simulink model "auv_modell_camsim_kalman"  (Simulink 7.0)
settings: Solver=ode4  StartTime=0.0  StopTime=100  FixedStep=0.1  RelTol=1e-3
values from neighbouring files (symbols this model uses):
  eta0 = [0 0 0 0 0 0]'    [initauv.m]
undefined symbols (not defined in the file or in its folder): C_calc, ekf
libraries: marine_gnc x2, fordypningsprosjekt x1, simulink x1
settings Model: Creator=anderga  LastModifiedBy=anderga  ExtModeAutoUpdateStatusClock=off  BufferReuse=off
settings OptimizationCC: BlockReduction=off  InlineParams=on  BufferReuse=off

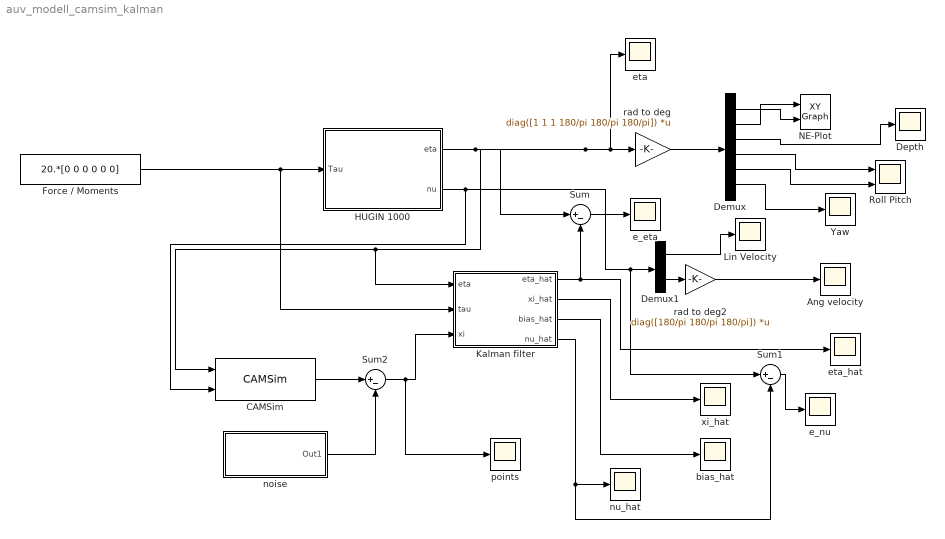
== system auv_modell_camsim_kalman ==
  Ang velocity : Scope
      settings: YMin=-1  YMax=1  SaveName=ScopeData6
  CAMSim : fordypningsprosjekt/CAMSim  SystemSampleTime=-1
  Demux : Demux  Outputs=6
  Demux1 : Demux  Outputs=2
  Depth : Scope
      settings: TimeRange=400  YMin=-140  YMax=40  SaveName=ScopeData4
  Force / Moments : Constant  Value=20.*[0 0 0 0 0 0]  OutDataType=sfix(16)  OutScaling=2^0
  HUGIN 1000 : Subsystem  mask(HUGIN 1000 AUV){eta_0=eta0, nu_0=[0 0 0 0 0 0]}
      mask prompts: eta_0 "Initial Position [x y z phi theta psi]"; nu_0 "Initial speed [u v w p q r]"
      mask help:
      | The hydrodynamic model of Kongsberg Maritimes
      | AUV type HUGIN 1000.
      |
      | Implemented using
      |
      | eta_dot = J(eta)*nu
      | M*nu_dot + C(nu)*nu + D(nu)*nu + g(eta) = tau
      |
      | and the MMS toolbox from www.marinecybernetics.org
      mask init:
      | m = 1380;
      | xg = 0;
      | yg = 0;
      | zg = 0.0328;
      | Ix = 86.53;
      | Iy = 1247;
      | Iz = 1247;
      | 
      | Xu = -85.57;
      | Yv = -1092.9;
      | Yr = -84.1448;
      | Zw = -1092.9;
      | Zq = 84.1448;
      | Mq = -795.1686;
      | Nr = -795.1686;
      |     
      | M = [m-Xu   0       0       0       m*zg    -m*yg;
      |      0      m-Yv    0       -m*zg   0       m*xg-Yr;
      |      0      0       m-Zw    m*yg    -m*xg-Zq 0;
      |      0      -m*zg   m*yg    Ix      0        0;
      |      m*zg   0       -m*xg-Zq 0      Iy-Mq    0;
      |      -m*yg  m*xg-Yr 0       0       0       Iz-Nr];
  Kalman filter : Subsystem
  Lin Velocity : Scope
      settings: YMin=-0.05  YMax=0.65
  NE-Plot : simulink/Sinks/XY Graph  SystemSampleTime=-1  xmin=-100  xmax=220  ymin=-100  ymax=1000  st=-1
  Roll Pitch : Scope  NumInputPorts=2
      settings: TimeRange=400  YMin=-1~-0.25  YMax=1~0  SaveName=ScopeData3
  Sum : Sum  Inputs=|+-  OutDataType=sfix(16)  OutScaling=2^0
  Sum1 : Sum  Inputs=|+-  OutDataType=sfix(16)  OutScaling=2^0
  Sum2 : Sum  Inputs=|+-  OutDataType=sfix(16)  OutScaling=2^0
  Yaw : Scope
      settings: TimeRange=100  YMin=1  YMax=4.75  SaveName=ScopeData2
  bias_hat : Scope
      settings: YMin=-0.015  YMax=0.001  SaveName=ScopeData11
  e_eta : Scope
      settings: TimeRange=100  YMin=-0.0007  YMax=5e-005  SaveName=ScopeData14
  e_nu : Scope
      settings: YMin=-0.25  YMax=2.75  SaveName=ScopeData15
  eta : Scope
      settings: YMax=6
  eta_hat : Scope
      settings: YMin=-80  YMax=10  SaveName=ScopeData9
  noise : Subsystem
  nu_hat : Scope
      settings: YMin=-200  YMax=25  SaveName=ScopeData12
  points : Scope
      settings: TimeRange=100  YMin=-7  YMax=7  SaveName=ScopeData13
  rad to deg : Gain  Gain=diag([1 1 1 180/pi 180/pi 180/pi])  Multiplication=Matrix(K*u)  ParameterDataType=sfix(16)  ParameterScaling=2^0  OutDataType=sfix(16)  OutScaling=2^0
  rad to deg2 : Gain  Gain=diag([180/pi 180/pi 180/pi])  Multiplication=Matrix(K*u)  ParameterDataType=sfix(16)  ParameterScaling=2^0  OutDataType=sfix(16)  OutScaling=2^0
  xi_hat : Scope
      settings: YMin=-4.5  YMax=1  SaveName=ScopeData10
  wires:
  Force / Moments/1 -> HUGIN 1000/1(Tau), Kalman filter/2(tau)
  HUGIN 1000/1(eta) -> eta/1, rad to deg/1, Sum/1, Kalman filter/1(eta), CAMSim/1
  Demux/2 -> NE-Plot/1
  Demux/1 -> NE-Plot/2
  Demux/6 -> Yaw/1
  Demux/4 -> Roll Pitch/1
  Demux/5 -> Roll Pitch/2
  Demux/3 -> Depth/1
  Demux1/1 -> Lin Velocity/1
  Demux1/2 -> rad to deg2/1
  HUGIN 1000/2(nu) -> Demux1/1, Sum1/1, CAMSim/2
  rad to deg/1 -> Demux/1
  rad to deg2/1 -> Ang velocity/1
  Kalman filter/1(eta_hat) -> eta_hat/1, Sum/2
  Kalman filter/2(xi_hat) -> xi_hat/1
  Kalman filter/3(bias_hat) -> bias_hat/1
  Kalman filter/4(nu_hat) -> nu_hat/1, Sum1/2
  Sum/1 -> e_eta/1
  Sum1/1 -> e_nu/1
  CAMSim/1 -> Sum2/1
  noise/1(Out1) -> Sum2/2
  Sum2/1 -> Kalman filter/3(xi), points/1

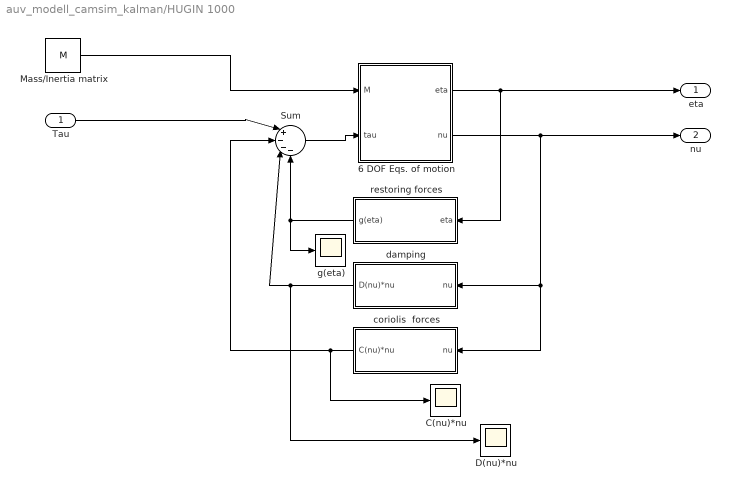
== system auv_modell_camsim_kalman/HUGIN 1000 ==
  Tau : Inport  OutDataType=sfix(16)  OutScaling=2^0
  6 DOF Eqs. of motion : Subsystem  AncestorBlock=marine_gnc/Models/ Kinetics /6 DOF Eqs. of motion  mask(Equations of motion){nu0=nu_0, eta0=eta_0}
      mask prompts: nu0 "Initial velocities (u,v,w,p,q,r)"; eta0 "Initial position/attitude (x,y,z,phi,theta,psi)"
      mask help:
      | 6 DOF equations of motion (surge, sway, heave, roll, pitch and yaw)
      |
      |    eta_dot = J(eta)*nu
      |    (M_RB+M_A)*nu_dot  =  tau
      |
      | where nu = [u,v,w,p,q,r]'  and eta = [x,y,z,phi,theta,psi]'
      |
      | T. I. Fossen (2002). Marine Control Systems: Guidance, Navigation and Control of Ships, Rigs and Underwater Vehicles, Marine Cybernetics AS, ISBN 82-92356-00-2
      |
      | Modified by Anders Garmo (2008)
  C(nu)*nu : Scope
      settings: TimeRange=100  YMin=-0.1  YMax=1.2  SaveName=ScopeData5
  D(nu)*nu : Scope
      settings: TimeRange=100  YMin=-10  YMax=100  SaveName=ScopeData8
  Mass/Inertia matrix : Constant  Value=M  OutDataType=sfix(16)  OutScaling=2^0
  Sum : Sum  Inputs=|+---  OutDataType=sfix(16)  OutScaling=2^0
  coriolis  forces : Subsystem  Orientation=left
      mask init:
      | W = 1380*9.81;
      | 
      | zg = 0.0328;
  damping : Subsystem  Orientation=left
      mask init:
      | Xu = -19.1881;
      | Yv = -931.9715;
      | Yr = 1915.8;
      | Zw = -931.9715;
      | Zq = -1915.8;
      | Kp = -1000;
      | Mw = 1760.7;
      | Mq = -8386.3;
      | Nv = -1760.7;
      | Nr = -8386.3;
      | 
      | Xuu = -3.8938;
      | 
      | D = [Xu 0 0 0 0 0;
      |       0 Yv 0 0 0 Yr;
      |       0 0 Zw 0 Zq 0;
      |       0 0 0 Kp 0 0;
      |       0 0 Mw 0 Mq 0;
      |       0 Nv 0 0 0 Nr];
  g(eta) : Scope
      settings: TimeRange=100  YMin=0  YMax=100  SaveName=ScopeData7
  restoring forces : Subsystem  Orientation=left
      mask init:
      | W = 1380*9.81;
      | 
      | zg = 0.0328;
  eta : Outport  OutDataType=sfix(16)  OutScaling=2^0
  nu : Outport  Port=2  OutDataType=sfix(16)  OutScaling=2^0
  wires:
  Mass/Inertia matrix/1 -> 6 DOF Eqs. of motion/1(M)
  6 DOF Eqs. of motion/2(nu) -> nu/1, damping/1(nu), coriolis  forces/1(nu)
  6 DOF Eqs. of motion/1(eta) -> restoring forces/1(eta), eta/1
  Sum/1 -> 6 DOF Eqs. of motion/2(tau)
  Tau/1 -> Sum/1
  coriolis  forces/1(C(nu)*nu) -> C(nu)*nu/1, Sum/2
  restoring forces/1(g(eta)) -> Sum/4, g(eta)/1
  damping/1(D(nu)*nu) -> Sum/3, D(nu)*nu/1

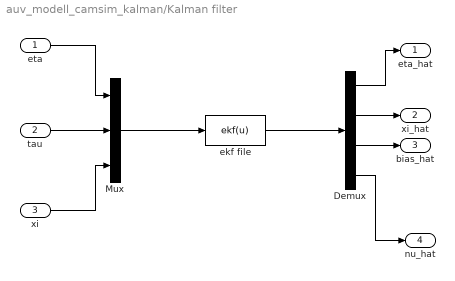
== system auv_modell_camsim_kalman/Kalman filter ==
  eta : Inport  OutDataType=sfix(16)  OutScaling=2^0
  tau : Inport  Port=2  OutDataType=sfix(16)  OutScaling=2^0
  xi : Inport  Port=3  OutDataType=sfix(16)  OutScaling=2^0
  Demux : Demux
  Mux : Mux  Inputs=3
  ekf file : MATLABFcn  MATLABFcn=ekf(u)  OutputDimensions=24
  eta_hat : Outport  OutDataType=sfix(16)  OutScaling=2^0
  xi_hat : Outport  Port=2  OutDataType=sfix(16)  OutScaling=2^0
  bias_hat : Outport  Port=3  OutDataType=sfix(16)  OutScaling=2^0
  nu_hat : Outport  Port=4  OutDataType=sfix(16)  OutScaling=2^0
  wires:
  eta/1 -> Mux/1
  tau/1 -> Mux/2
  xi/1 -> Mux/3
  Demux/1 -> eta_hat/1
  Demux/2 -> xi_hat/1
  Demux/3 -> bias_hat/1
  Demux/4 -> nu_hat/1
  Mux/1 -> ekf file/1
  ekf file/1 -> Demux/1

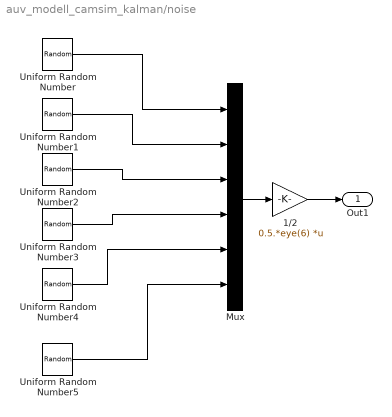
== system auv_modell_camsim_kalman/noise ==
  1/2 : Gain  Gain=0.5.*eye(6)  Multiplication=Matrix(K*u)  ParameterDataType=sfix(16)  ParameterScaling=2^0  OutDataType=sfix(16)  OutScaling=2^0
  Mux : Mux  Inputs=6
  Uniform Random Number : UniformRandomNumber  Seed=15  SampleTime=0
  Uniform Random Number1 : UniformRandomNumber  Seed=16  SampleTime=0
  Uniform Random Number2 : UniformRandomNumber  Seed=17  SampleTime=0
  Uniform Random Number3 : UniformRandomNumber  Seed=18  SampleTime=0
  Uniform Random Number4 : UniformRandomNumber  Seed=19  SampleTime=0
  Uniform Random Number5 : UniformRandomNumber  Seed=20  SampleTime=0
  Out1 : Outport  OutDataType=sfix(16)  OutScaling=2^0
  wires:
  Mux/1 -> 1/2/1
  Uniform Random Number5/1 -> Mux/6
  Uniform Random Number4/1 -> Mux/5
  Uniform Random Number3/1 -> Mux/4
  Uniform Random Number2/1 -> Mux/3
  Uniform Random Number1/1 -> Mux/2
  Uniform Random Number/1 -> Mux/1
  1/2/1 -> Out1/1

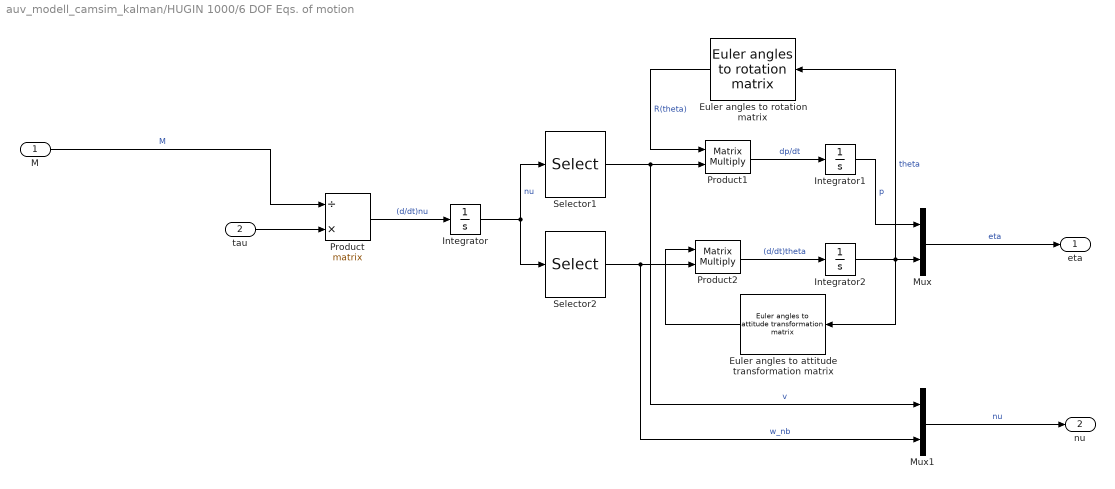
== system auv_modell_camsim_kalman/HUGIN 1000/6 DOF Eqs. of motion ==
  M : Inport  OutDataType=sfix(16)  OutScaling=2^0
  tau : Inport  Port=2  OutDataType=sfix(16)  OutScaling=2^0
  Euler angles to rotation matrix : marine_gnc/Models/ Kinematics/Euler angles to rotation matrix  Orientation=left  SystemSampleTime=-1
  Euler angles to attitude transformation matrix : marine_gnc/Models/ Kinematics/Euler angles to attitude transformation matrix  Orientation=left  SystemSampleTime=-1
  Integrator : Integrator  InitialCondition=nu0
  Integrator1 : Integrator  InitialCondition=eta0(1:3)
  Integrator2 : Integrator  InitialCondition=eta0(4:6)
  Mux : Mux  Inputs=2
  Mux1 : Mux  Inputs=2
  Product : Product  Inputs=/*  Multiplication=Matrix(*)  OutDataType=sfix(16)  OutScaling=2^0  SaturateOnIntegerOverflow=on
  Product1 : Product  Inputs=**  Multiplication=Matrix(*)  OutDataType=sfix(16)  OutScaling=2^0  SaturateOnIntegerOverflow=on
  Product2 : Product  Inputs=**  Multiplication=Matrix(*)  OutDataType=sfix(16)  OutScaling=2^0  SaturateOnIntegerOverflow=on
  Selector1 : Selector  InputPortWidth=6  IndexOptions=Index vector (dialog)  Indices=[1 2 3]  OutputSizes=1
  Selector2 : Selector  InputPortWidth=6  IndexOptions=Index vector (dialog)  Indices=[4 5 6]  OutputSizes=1
  eta : Outport  OutDataType=sfix(16)  OutScaling=2^0
  nu : Outport  Port=2  OutDataType=sfix(16)  OutScaling=2^0
  wires:
  tau/1 -> Product/2
  Euler angles to attitude transformation matrix/1 -> Product2/1
  Mux1/1 -> nu/1  "nu"
  Mux/1 -> eta/1  "eta"
  Integrator1/1 -> Mux/1  "p"
  Integrator2/1 -> Euler angles to attitude transformation matrix/1, Euler angles to rotation matrix/1, Mux/2  "theta"
  Product2/1 -> Integrator2/1  "(d/dt)theta"
  Euler angles to rotation matrix/1 -> Product1/1  "R(theta)"
  Product1/1 -> Integrator1/1  "dp/dt"
  Selector2/1 -> Product2/2, Mux1/2  "w_nb"
  Selector1/1 -> Mux1/1, Product1/2  "v"
  Integrator/1 -> Selector2/1, Selector1/1  "nu"
  Product/1 -> Integrator/1  "(d/dt)nu"
  M/1 -> Product/1  "M"

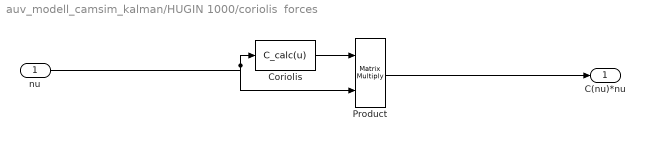
== system auv_modell_camsim_kalman/HUGIN 1000/coriolis  forces ==
  nu : Inport  OutDataType=sfix(16)  OutScaling=2^0
  Coriolis : MATLABFcn  MATLABFcn=C_calc(u)  OutputDimensions=[6,6]  Output1D=off
  Product : Product  Multiplication=Matrix(*)  OutDataType=sfix(16)  OutScaling=2^0  RndMeth=Zero
  C(nu)*nu : Outport  OutDataType=sfix(16)  OutScaling=2^0
  wires:
  nu/1 -> Product/2, Coriolis/1
  Coriolis/1 -> Product/1
  Product/1 -> C(nu)*nu/1

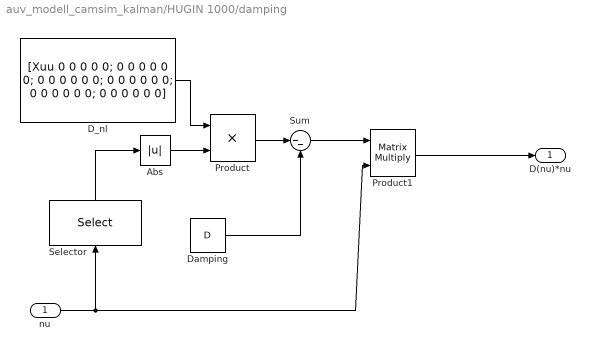
== system auv_modell_camsim_kalman/HUGIN 1000/damping ==
  nu : Inport  OutDataType=sfix(16)  OutScaling=2^0
  Abs : Abs  OutDataType=sfix(16)  OutScaling=2^0
  D_nl : Constant  Value=[Xuu 0 0 0 0 0; 0 0 0 0 0 0; 0 0 0 0 0 0; 0 0 0 0 0 0; 0 0 0 0 0 0; 0 0 0 0 0 0]  OutDataType=sfix(16)  OutScaling=2^0
  Damping : Constant  Value=D  OutDataType=sfix(16)  OutScaling=2^0
  Product : Product  OutDataType=sfix(16)  OutScaling=2^0  RndMeth=Zero
  Product1 : Product  Multiplication=Matrix(*)  OutDataType=sfix(16)  OutScaling=2^0  RndMeth=Zero
  Selector : Selector  Orientation=up  InputPortWidth=6  IndexOptions=Index vector (dialog)  Indices=[1]  OutputSizes=1
  Sum : Sum  Inputs=|--  OutDataType=sfix(16)  OutScaling=2^0
  D(nu)*nu : Outport  OutDataType=sfix(16)  OutScaling=2^0
  wires:
  Damping/1 -> Sum/2
  Product/1 -> Sum/1
  nu/1 -> Product1/2, Selector/1
  D_nl/1 -> Product/1
  Abs/1 -> Product/2
  Sum/1 -> Product1/1
  Product1/1 -> D(nu)*nu/1
  Selector/1 -> Abs/1

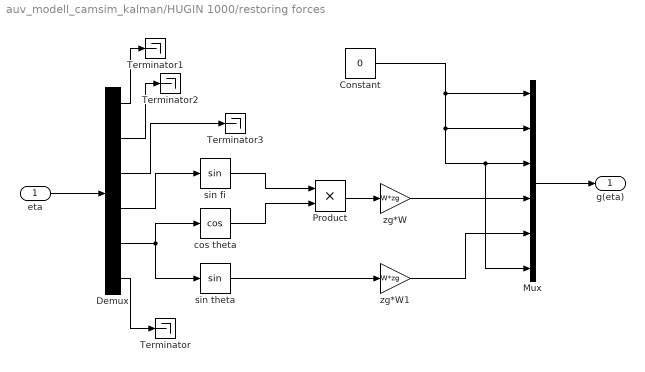
== system auv_modell_camsim_kalman/HUGIN 1000/restoring forces ==
  eta : Inport  OutDataType=sfix(16)  OutScaling=2^0
  Constant : Constant  Value=0  OutDataType=sfix(16)  OutScaling=2^0
  Demux : Demux  Outputs=6
  Mux : Mux  Inputs=6
  Product : Product  OutDataType=sfix(16)  OutScaling=2^0  RndMeth=Zero
  Terminator{,1..3} (4 alike) : Terminator
  cos theta : Trigonometry  Operator=cos
  sin fi : Trigonometry
  sin theta : Trigonometry
  zg*W : Gain  Gain=W*zg  ParameterDataType=sfix(16)  ParameterScaling=2^0  OutDataType=sfix(16)  OutScaling=2^0
  zg*W1 : Gain  Gain=W*zg  ParameterDataType=sfix(16)  ParameterScaling=2^0  OutDataType=sfix(16)  OutScaling=2^0
  g(eta) : Outport  OutDataType=sfix(16)  OutScaling=2^0
  wires:
  eta/1 -> Demux/1
  Demux/4 -> sin fi/1
  Demux/5 -> cos theta/1, sin theta/1
  cos theta/1 -> Product/2
  sin fi/1 -> Product/1
  Product/1 -> zg*W/1
  sin theta/1 -> zg*W1/1
  Mux/1 -> g(eta)/1
  zg*W1/1 -> Mux/5
  zg*W/1 -> Mux/4
  Constant/1 -> Mux/1, Mux/2, Mux/3, Mux/6
  Demux/6 -> Terminator/1
  Demux/1 -> Terminator1/1
  Demux/2 -> Terminator2/1
  Demux/3 -> Terminator3/1
